simulink model "Pid_Fuzzy_Carro_pendulo"  (R2016a)
settings: Solver=ode3  StartTime=0.0  StopTime=inf  FixedStep=h  RelTol=1e-3
values from neighbouring files (symbols this model uses):
  h = 0.001    [Constantes.m]
undefined symbols (not defined in the file or in its folder): National_Instruments, PCI
libraries: sldrtlib x4, fuzblock x1
settings Model: SimulationMode=external  Creator=Jovani  LastModifiedBy=MCAC-UAEH
settings DataIOCC: LimitDataPoints=on  SaveFormat=Array
settings DebuggingCC: UnderspecifiedInitializationDetection=Classic  MergeDetectMultiDrivingBlocksExec=none  SolverPrmCheckMsg=warning  StateNameClashWarn=warning
settings HardwareCC: ProdBitPerLong=64  ProdLargestAtomicFloat=None  ProdHWDeviceType=Intel->x86-64  TargetBitPerLong=64  TargetBitPerPointer=64  TargetIntDivRoundTo=Zero  TargetEndianess=LittleEndian  TargetWordSize=64  TargetHWDeviceType=Intel->x86-64
settings ModelReferenceCC: PropagateSignalLabelsOutOfModel=off
settings RTWCC: SystemTargetFile=sldrt.tlc  TemplateMakefile=sldrt.tmf  Description=Simulink Desktop Real-Time  RTWCompilerOptimization=on
settings CodeAppCC: MaxIdLength=95
settings SimulinkDesktopRealTimeCC: TargetPreCompLibLocation=C:\Program Files\MATLAB\R2016a\toolbox\sldrt\lib\win64  TargetLangStandard=C89/C90 (ANSI)  SupportVariableSizeSignals=off
settings ConfigComp: CovModelRefEnable=Off

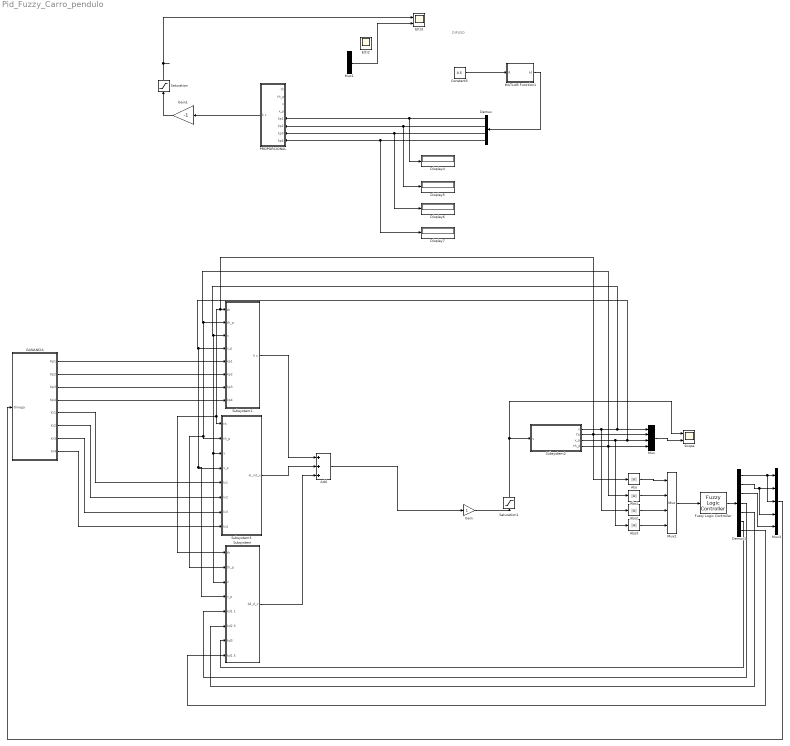
== system Pid_Fuzzy_Carro_pendulo ==
  note: DIFUSO
  Abs{,1..3} (4 alike) : Abs
  Add : Sum  Inputs=+++
  Constant5 : Constant  Value=0.5
  Demux : Demux
  Demux1 : Demux  Outputs=7
  Display{4..7} (4 alike) : Display
  E(t)2 : Scope  NumInputPorts=4
  E(t)3 : Scope  NumInputPorts=2
  Fuzzy Logic Controller : fuzblock/Fuzzy Logic  Controller  fis=pi_2
  GANANCIA : Subsystem
  Gain : Gain
  Gain1 : Gain  Gain=-1
  MATLAB Function1 : MATLAB Function  TreatAsAtomicUnit=on
  Mux : Mux
  Mux1 : Mux
  Mux2 : Mux
  Mux3 : Mux  Inputs=5
  PROPORCIONAL : Subsystem
  Saturation : Saturate  UpperLimit=7.5  LowerLimit=-7.5
  Saturation1 : Saturate  UpperLimit=7.5  LowerLimit=-7.5
  Scope : Scope  NumInputPorts=2
  Subsystem : Subsystem
  Subsystem1 : Subsystem
  Subsystem2 : Subsystem
  Subsystem3 : Subsystem
  wires:
  Gain1/1 -> Saturation/1
  ? -> PROPORCIONAL/2(th_p), Mux1/4, E(t)2/3
  ? -> E(t)2/4, Mux1/3, PROPORCIONAL/4(x_p)
  ? -> E(t)2/2, Mux1/2, PROPORCIONAL/1(th)
  ? -> E(t)2/1, Mux1/1, PROPORCIONAL/3(x)
  Mux1/1 -> E(t)3/2
  PROPORCIONAL/1(k x) -> Gain1/1
  Saturation/1 -> E(t)3/1
  Constant5/1 -> MATLAB Function1/1(R)
  MATLAB Function1/1(kf) -> Demux/1
  Demux/1 -> Display4/1, PROPORCIONAL/5(kp1)
  Demux/2 -> Display5/1, PROPORCIONAL/6(kp2)
  Demux/3 -> Display6/1, PROPORCIONAL/7(kp3)
  Demux/4 -> Display7/1, PROPORCIONAL/8(kp4)
  GANANCIA/1(Kp1) -> Subsystem1/5("kp1 ")
  GANANCIA/2(Kp2) -> Subsystem1/6(kp2)
  GANANCIA/3("Kp3 ") -> Subsystem1/7(kp3)
  GANANCIA/4(Kp4) -> Subsystem1/8(kp4)
  GANANCIA/5("Ki1 ") -> Subsystem3/5(ki1)
  GANANCIA/6("Ki2 ") -> Subsystem3/6(ki2)
  GANANCIA/7("Ki3 ") -> Subsystem3/7(ki3)
  GANANCIA/8("Ki4 ") -> Subsystem3/8(ki4)
  Mux/1 -> Scope/2
  Gain/1 -> Saturation1/1
  Add/1 -> Gain/1
  Subsystem1/1(k x) -> Add/1
  Subsystem3/1(ki_int_x) -> Add/2
  Subsystem/1("kd_d_x ") -> Add/3
  Subsystem2/1(x) -> Abs2/1, Subsystem/3("x "), Subsystem3/3(x), Subsystem1/3(x), Mux/1
  Subsystem2/3(x_p) -> Abs3/1, Subsystem/4("x_p "), Subsystem3/4(x_p), Subsystem1/4(x_p), Mux/3
  Subsystem2/2(Th) -> Abs/1, Subsystem/1("th "), Subsystem3/1("th "), Subsystem1/1("th "), Mux/2
  Subsystem2/4(th_p) -> Abs1/1, Subsystem/2("th_p "), Subsystem3/2(th_p), Subsystem1/2(th_p), Mux/4
  Abs/1 -> Mux2/1
  Abs1/1 -> Mux2/2
  Abs2/1 -> Mux2/3
  Abs3/1 -> Mux2/4
  Mux2/1 -> Fuzzy Logic Controller/1
  Fuzzy Logic Controller/1 -> Demux1/1
  Demux1/1 -> Mux3/3, Mux3/1
  Demux1/2 -> Mux3/4, Mux3/2
  Demux1/3 -> Mux3/5
  Demux1/4 -> Subsystem/5(kd1 1)
  Demux1/5 -> Subsystem/6(kd2 3)
  Demux1/6 -> Subsystem/7("kd3 ")
  Demux1/7 -> Subsystem/8(kd1 5)
  Mux3/1 -> GANANCIA/1(Omega)
  Saturation1/1 -> Subsystem2/1(u), Scope/1
  ? -> ?

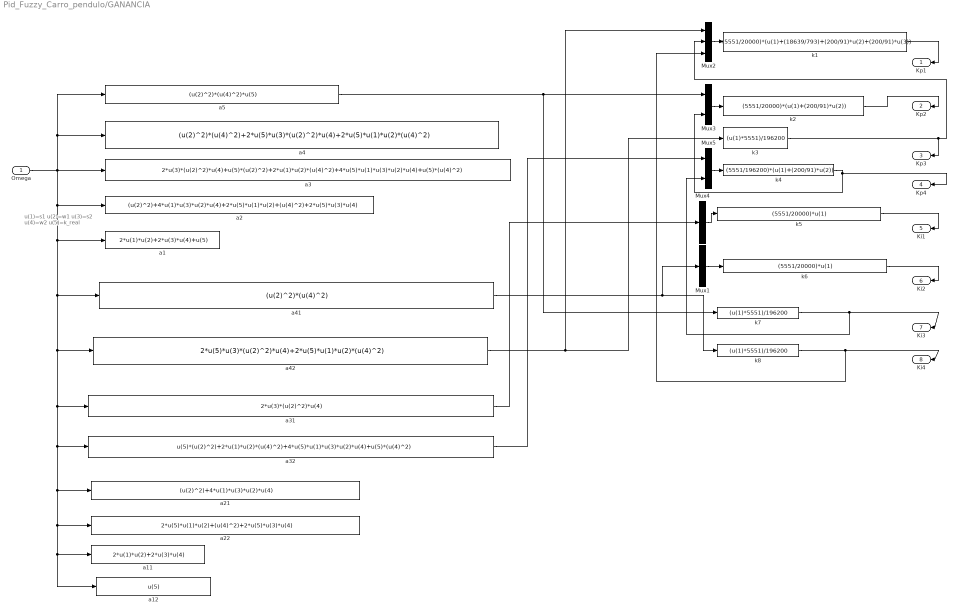
== system Pid_Fuzzy_Carro_pendulo/GANANCIA ==
  note: u(1)=s1
      | u(2)=w1
      | u(3)=s2
      | u(4)=w2
      | u(5)=k_real
  Omega : Inport
  Mux1 : Mux  Inputs=1
  Mux2 : Mux  Inputs=3
  Mux3 : Mux  Inputs=2
  Mux4 : Mux  Inputs=1
  Mux5 : Mux  Inputs=2
  "a1 " : Fcn  Expr=2*u(1)*u(2)+2*u(3)*u(4)+u(5)
  "a11 " : Fcn  Expr=2*u(1)*u(2)+2*u(3)*u(4)
  a12 : Fcn  Expr=u(5)
  "a2 " : Fcn  Expr=(u(2)^2)+4*u(1)*u(3)*u(2)*u(4)+2*u(5)*u(1)*u(2)+(u(4)^2)+2*u(5)*u(3)*u(4)
  "a21 " : Fcn  Expr=(u(2)^2)+4*u(1)*u(3)*u(2)*u(4)
  "a22 " : Fcn  Expr=2*u(5)*u(1)*u(2)+(u(4)^2)+2*u(5)*u(3)*u(4)
  a3 : Fcn  Expr=2*u(3)*(u(2)^2)*u(4)+u(5)*(u(2)^2)+2*u(1)*u(2)*(u(4)^2)+4*u(5)*u(1)*u(3)*u(2)*u(4)+u(5)*(u(4)^2)
  a31 : Fcn  Expr=2*u(3)*(u(2)^2)*u(4)
  a32 : Fcn  Expr=u(5)*(u(2)^2)+2*u(1)*u(2)*(u(4)^2)+4*u(5)*u(1)*u(3)*u(2)*u(4)+u(5)*(u(4)^2)
  a4 : Fcn  Expr=(u(2)^2)*(u(4)^2)+2*u(5)*u(3)*(u(2)^2)*u(4)+2*u(5)*u(1)*u(2)*(u(4)^2)
  a41 : Fcn  Expr=(u(2)^2)*(u(4)^2)
  a42 : Fcn  Expr=2*u(5)*u(3)*(u(2)^2)*u(4)+2*u(5)*u(1)*u(2)*(u(4)^2)
  a5 : Fcn  Expr=(u(2)^2)*(u(4)^2)*u(5)
  k1 : Fcn  Expr=(5551/20000)*(u(1)+(18639/793)+(200/91)*u(2)+(200/91)*u(3))
  k2 : Fcn  Expr=(5551/20000)*(u(1)+(200/91)*u(2))
  k3 : Fcn  Expr=(u(1)*5551)/196200
  k4 : Fcn  Expr=(5551/196200)*(u(1)+(200/91)*u(2))
  "k5 " : Fcn  Expr=(5551/20000)*u(1)
  "k6 " : Fcn  Expr=(5551/20000)*u(1)
  k7 : Fcn  Expr=(u(1)*5551)/196200
  k8 : Fcn  Expr=(u(1)*5551)/196200
  Kp1 : Outport
  Kp2 : Outport  Port=2
  "Kp3 " : Outport  Port=3
  Kp4 : Outport  Port=4
  "Ki1 " : Outport  Port=5
  "Ki2 " : Outport  Port=6
  "Ki3 " : Outport  Port=7
  "Ki4 " : Outport  Port=8
  wires:
  a32/1 -> Mux5/1
  Mux5/1 -> k4/1
  Mux1/1 -> "k6 "/1
  "k6 "/1 -> "Ki2 "/1
  a31/1 -> Mux4/1
  a41/1 -> k8/1, Mux1/1
  a42/1 -> k3/1, Mux2/1
  k2/1 -> Kp2/1
  k1/1 -> Kp1/1
  Mux3/1 -> k2/1
  Mux2/1 -> k1/1
  k4/1 -> Kp4/1, Mux3/2
  "k5 "/1 -> "Ki1 "/1
  k8/1 -> "Ki4 "/1, Mux2/3
  k3/1 -> "Kp3 "/1, Mux2/2
  a5/1 -> Mux3/1, k7/1
  k7/1 -> "Ki3 "/1, Mux5/2
  Omega/1 -> a4/1, a5/1, a3/1, "a2 "/1, "a1 "/1, a41/1, a42/1, a31/1, a32/1, "a21 "/1, "a22 "/1, "a11 "/1, a12/1
  Mux4/1 -> "k5 "/1

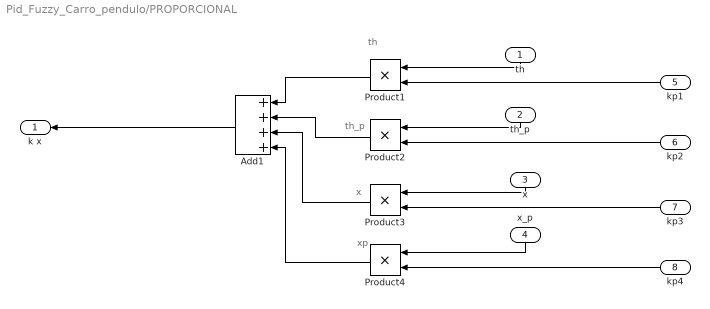
== system Pid_Fuzzy_Carro_pendulo/PROPORCIONAL ==
  note: xp
  note: x
  note: th_p
  note: th
  th : Inport
  th_p : Inport  Port=2
  x : Inport  Port=3
  x_p : Inport  Port=4
  kp1 : Inport  Port=5
  kp2 : Inport  Port=6
  kp3 : Inport  Port=7
  kp4 : Inport  Port=8
  Add1 : Sum  Inputs=++++
  Product{1..4} (4 alike) : Product
  k x : Outport
  wires:
  x_p/1 -> Product4/1
  x/1 -> Product3/1
  th_p/1 -> Product2/1
  th/1 -> Product1/1
  Add1/1 -> k x/1
  Product4/1 -> Add1/4
  Product3/1 -> Add1/3
  Product2/1 -> Add1/2
  Product1/1 -> Add1/1
  kp3/1 -> Product3/2
  kp1/1 -> Product1/2
  kp2/1 -> Product2/2
  kp4/1 -> Product4/2

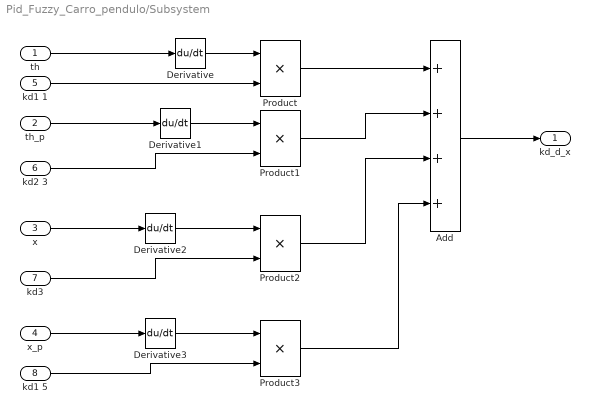
== system Pid_Fuzzy_Carro_pendulo/Subsystem ==
  "th " : Inport
  "th_p " : Inport  Port=2
  "x " : Inport  Port=3
  "x_p " : Inport  Port=4
  kd1 1 : Inport  Port=5
  kd2 3 : Inport  Port=6
  "kd3 " : Inport  Port=7
  kd1 5 : Inport  Port=8
  Add : Sum  Inputs=++++
  Derivative{,1..3} (4 alike) : Derivative
  Product{,1..3} (4 alike) : Product
  "kd_d_x " : Outport
  wires:
  Derivative/1 -> Product/1
  Derivative1/1 -> Product1/1
  Product2/1 -> Add/3
  kd1 1/1 -> Product/2
  Product3/1 -> Add/4
  Product1/1 -> Add/2
  Add/1 -> "kd_d_x "/1
  kd1 5/1 -> Product3/2
  kd2 3/1 -> Product1/2
  Derivative3/1 -> Product3/1
  Product/1 -> Add/1
  "x "/1 -> Derivative2/1
  "x_p "/1 -> Derivative3/1
  "th_p "/1 -> Derivative1/1
  Derivative2/1 -> Product2/1
  "kd3 "/1 -> Product2/2
  "th "/1 -> Derivative/1

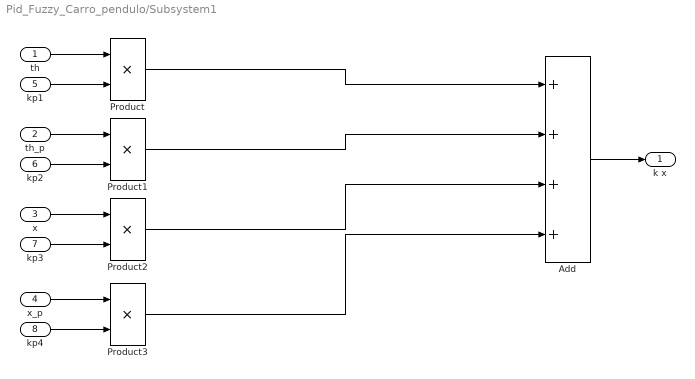
== system Pid_Fuzzy_Carro_pendulo/Subsystem1 ==
  "th " : Inport
  th_p : Inport  Port=2
  x : Inport  Port=3
  x_p : Inport  Port=4
  "kp1 " : Inport  Port=5
  kp2 : Inport  Port=6
  kp3 : Inport  Port=7
  kp4 : Inport  Port=8
  Add : Sum  Inputs=++++
  Product{,1..3} (4 alike) : Product
  k x : Outport
  wires:
  th_p/1 -> Product1/1
  "th "/1 -> Product/1
  x/1 -> Product2/1
  "kp1 "/1 -> Product/2
  kp4/1 -> Product3/2
  Product2/1 -> Add/3
  x_p/1 -> Product3/1
  Product3/1 -> Add/4
  kp2/1 -> Product1/2
  kp3/1 -> Product2/2
  Add/1 -> k x/1
  Product/1 -> Add/1
  Product1/1 -> Add/2

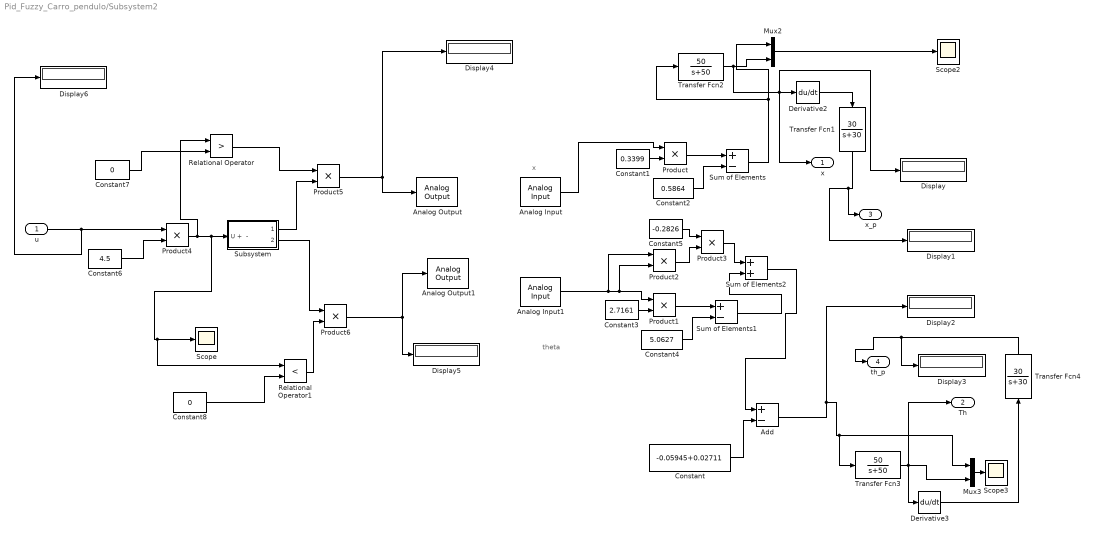
== system Pid_Fuzzy_Carro_pendulo/Subsystem2 ==
  note: x
  note: theta
  u : Inport
  Add : Sum  Inputs=+-
  Analog Input : sldrtlib/Analog Input  SampleTime=h  MaxMissedTicks=10  ShowMissedTicks=off  YieldWhenWaiting=off  DrvName=National_Instruments/PCI-6071E  DrvAddress=0  DrvOptions=[0 0 0 0 0 0]  Channels=9  RangeMode=1  VoltRange=10  DataType=1
      settings: AttributesFormatString=National Instruments\nPCI-6071E [0h]
  Analog Input1 : sldrtlib/Analog Input  SampleTime=h  MaxMissedTicks=10  ShowMissedTicks=off  YieldWhenWaiting=off  DrvName=National_Instruments/PCI-6071E  DrvAddress=0  DrvOptions=[0 0 0 0 0 0]  Channels=2  RangeMode=1  VoltRange=10  DataType=1
      settings: AttributesFormatString=National Instruments\nPCI-6071E [0h]
  Analog Output : sldrtlib/Analog Output  SampleTime=h  MaxMissedTicks=10  ShowMissedTicks=off  YieldWhenWaiting=off  DrvName=National_Instruments/PCI-6071E  DrvAddress=0  DrvOptions=[0 0 0 0 0 0]  Channels=1  RangeMode=1  VoltRange=1  InitialValue=[]  FinalValue=[]
      settings: AttributesFormatString=National Instruments\nPCI-6071E [0h]
  Analog Output1 : sldrtlib/Analog Output  SampleTime=h  MaxMissedTicks=10  ShowMissedTicks=off  YieldWhenWaiting=off  DrvName=National_Instruments/PCI-6071E  DrvAddress=0  DrvOptions=[0 0 0 0 0 0]  Channels=2  RangeMode=1  VoltRange=1  InitialValue=[]  FinalValue=[]
      settings: AttributesFormatString=National Instruments\nPCI-6071E [0h]
  Constant : Constant  Value=-0.05945+0.02711
  Constant1 : Constant  Value=0.3399
  Constant2 : Constant  Value=0.5864
  Constant3 : Constant  Value=2.7161
  Constant4 : Constant  Value=5.0627
  Constant5 : Constant  Value=-0.2826
  Constant6 : Constant  Value=4.5
  Constant7 : Constant  Value=0
  Constant8 : Constant  Value=0
  Derivative2 : Derivative
  Derivative3 : Derivative
  Display{,1..6} (7 alike) : Display
  Mux2 : Mux  Inputs=2
  Mux3 : Mux  Inputs=2
  Product{,1..6} (7 alike) : Product
  Relational Operator : RelationalOperator  Operator=>  OutDataTypeStr=boolean
  Relational Operator1 : RelationalOperator  Operator=<  OutDataTypeStr=boolean
  Scope : Scope
  Scope2 : Scope
  Scope3 : Scope
  Subsystem : Subsystem
  Sum of Elements : Sum  Inputs=+-
  Sum of Elements1 : Sum  Inputs=+-
  Sum of Elements2 : Sum
  Transfer Fcn1 : TransferFcn  Numerator=[30]  Denominator=[1 30]
  Transfer Fcn2 : TransferFcn  Numerator=[50]  Denominator=[1 50]
  Transfer Fcn3 : TransferFcn  Numerator=[50]  Denominator=[1 50]
  Transfer Fcn4 : TransferFcn  Numerator=[30]  Denominator=[1 30]
  x : Outport
  Th : Outport  Port=2
  x_p : Outport  Port=3
  th_p : Outport  Port=4
  wires:
  Transfer Fcn4/1 -> th_p/1, Display3/1
  Transfer Fcn1/1 -> x_p/1, Display1/1
  Transfer Fcn3/1 -> Mux3/2, Derivative3/1, Th/1
  Mux3/1 -> Scope3/1
  Transfer Fcn2/1 -> Mux2/2, Derivative2/1, Display/1, x/1
  Mux2/1 -> Scope2/1
  Derivative3/1 -> Transfer Fcn4/1
  Derivative2/1 -> Transfer Fcn1/1
  Subsystem/2(neg ++) -> Product6/1
  Subsystem/1(pos ++) -> Product5/2
  Constant/1 -> Add/2
  Sum of Elements2/1 -> Add/1
  Relational Operator/1 -> Product5/1
  Product6/1 -> Analog Output1/1, Display5/1
  Relational Operator1/1 -> Product6/2
  Constant8/1 -> Relational Operator1/2
  Product5/1 -> Display4/1, Analog Output/1
  Constant7/1 -> Relational Operator/2
  Product4/1 -> Subsystem/1(U +  -), Scope/1, Relational Operator1/1, Relational Operator/1
  Constant6/1 -> Product4/2
  u/1 -> Product4/1, Display6/1
  Sum of Elements1/1 -> Sum of Elements2/2
  Product3/1 -> Sum of Elements2/1
  Product2/1 -> Product3/2
  Constant5/1 -> Product3/1
  Constant4/1 -> Sum of Elements1/2
  Constant3/1 -> Product1/2
  Product1/1 -> Sum of Elements1/1
  Sum of Elements/1 -> Transfer Fcn2/1, Mux2/1
  Constant2/1 -> Sum of Elements/2
  Constant1/1 -> Product/2
  Product/1 -> Sum of Elements/1
  Analog Input/1 -> Product/1
  Analog Input1/1 -> Product1/1, Product2/2, Product2/1
  Add/1 -> Mux3/1, Transfer Fcn3/1, Display2/1

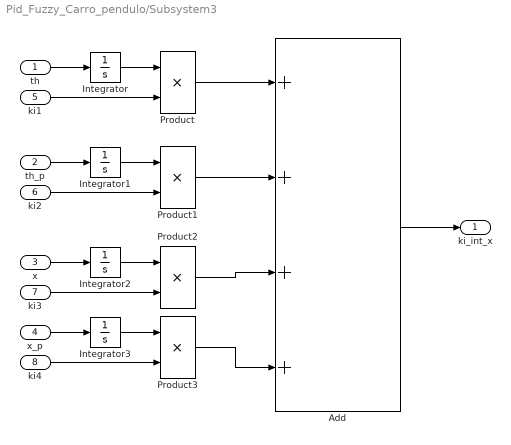
== system Pid_Fuzzy_Carro_pendulo/Subsystem3 ==
  "th " : Inport
  th_p : Inport  Port=2
  x : Inport  Port=3
  x_p : Inport  Port=4
  ki1 : Inport  Port=5
  ki2 : Inport  Port=6
  ki3 : Inport  Port=7
  ki4 : Inport  Port=8
  Add : Sum  Inputs=++++
  Integrator{,1..3} (4 alike) : Integrator
  Product{,1..3} (4 alike) : Product
  ki_int_x : Outport
  wires:
  Product3/1 -> Add/4
  Product2/1 -> Add/3
  Product/1 -> Add/1
  Integrator3/1 -> Product3/1
  "th "/1 -> Integrator/1
  ki1/1 -> Product/2
  ki2/1 -> Product1/2
  ki3/1 -> Product2/2
  ki4/1 -> Product3/2
  Product1/1 -> Add/2
  th_p/1 -> Integrator1/1
  Integrator1/1 -> Product1/1
  x_p/1 -> Integrator3/1
  Integrator2/1 -> Product2/1
  x/1 -> Integrator2/1
  Integrator/1 -> Product/1
  Add/1 -> ki_int_x/1

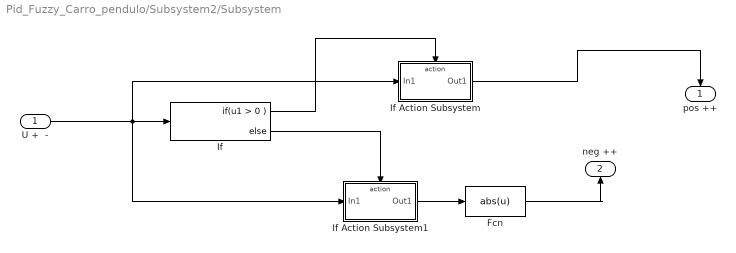
== system Pid_Fuzzy_Carro_pendulo/Subsystem2/Subsystem ==
  U +  - : Inport
  Fcn : Fcn  Expr=abs(u)
  If : If  IfExpression=u1 > 0
  If Action Subsystem : Subsystem  TreatAsAtomicUnit=on
  If Action Subsystem1 : Subsystem  TreatAsAtomicUnit=on
  pos ++ : Outport
  neg ++ : Outport  Port=2
  wires:
  Fcn/1 -> neg ++/1
  If Action Subsystem1/1(Out1) -> Fcn/1
  If Action Subsystem/1(Out1) -> pos ++/1
  If/2 -> If Action Subsystem1/Action
  U +  -/1 -> If/1, If Action Subsystem/1(In1), If Action Subsystem1/1(In1)
  If/1 -> If Action Subsystem/Action

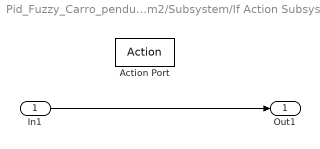
== system Pid_Fuzzy_Carro_pendulo/Subsystem2/Subsystem/If Action Subsystem ==
  In1 : Inport
  Action Port : ActionPort  ActionType=then
  Out1 : Outport
  wires:
  In1/1 -> Out1/1

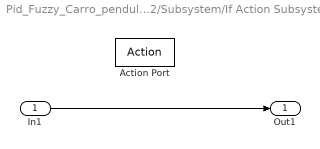
== system Pid_Fuzzy_Carro_pendulo/Subsystem2/Subsystem/If Action Subsystem1 ==
  In1 : Inport
  Action Port : ActionPort  ActionType=else
  Out1 : Outport
  wires:
  In1/1 -> Out1/1

== matlab function Pid_Fuzzy_Carro_pendulo/MATLAB Function1 ==
  data: R input; kf output
function kf = fcn(R)
%#codegen
%kf=[-60.1155,-15.6512,-6.3246,-10.4452];
kf=[-60.1155,-15.6512,-6.3246,-10.4452];

end
